simulink model "ros_image_filters_0619"  (R2017a)
settings: Solver=FixedStepDiscrete  StartTime=0.0  StopTime=inf  FixedStep=0.01  RelTol=1e-3  EnableMultiTasking=on
model workspace (MAT data in the model file):
  SL_ROS_VariableLengthArrays_MaxSizes.CommonInfo.ArrayTruncateAction = 'EmitWarning'
  SL_ROS_VariableLengthArrays_MaxSizes.MsgTypeMap = containers.Map
  SL_ROS_VariableLengthArrays_MaxSizes.MsgTypeMap.serialization.keys = {'sensor_msgs/Image'}
  SL_ROS_VariableLengthArrays_MaxSizes.MsgTypeMap.serialization.values{1}(1).PropertyName = 'Data'
  SL_ROS_VariableLengthArrays_MaxSizes.MsgTypeMap.serialization.values{1}(1).DataType = 'uint8'
  SL_ROS_VariableLengthArrays_MaxSizes.MsgTypeMap.serialization.values{1}(1).MaxLength = 1555200
  SL_ROS_VariableLengthArrays_MaxSizes.MsgTypeMap.serialization.values{1}(2).PropertyName = 'Encoding'
  SL_ROS_VariableLengthArrays_MaxSizes.MsgTypeMap.serialization.values{1}(2).DataType = 'uint8'
  SL_ROS_VariableLengthArrays_MaxSizes.MsgTypeMap.serialization.values{1}(2).MaxLength = 5
  SL_ROS_VariableLengthArrays_MaxSizes.MsgTypeMap.serialization.uniformity = 0
  SL_ROS_VariableLengthArrays_MaxSizes.MsgTypeMap.serialization.keyType = 'char'
  SL_ROS_VariableLengthArrays_MaxSizes.MsgTypeMap.serialization.valueType = 'any'
  blockSize = [270 480]
undefined symbols (not defined in the file): gray, M, N, Rec, SDTV, strel, sz
libraries: vipmisc x9, visionsinks x6, robotlib x5, visionconversions x4, simulink x3, visionanalysis x2, visionfilter x1, visionmorphops x1
settings Model: Creator=qifan  LastModifiedBy=qifan
settings SolverCC: AutoInsertRateTranBlk=on
settings DataIOCC: SaveOutput=off  SaveTime=off
settings OptimizationCC: PassReuseOutputArgsAs=Individual arguments  StateBitsets=on  DataBitsets=on  ZeroExternalMemoryAtStartup=off  ZeroInternalMemoryAtStartup=off  NoFixptDivByZeroProtection=on  LifeSpan=1  MaxStackSize=64
settings DebuggingCC: ParameterTunabilityLossMsg=error
settings HardwareCC: ProdBitPerPointer=32  ProdBitPerSizeT=32  ProdBitPerPtrDiffT=32  ProdLargestAtomicFloat=None  ProdIntDivRoundTo=Undefined  ProdEndianess=Unspecified  ProdWordSize=32  ProdHWDeviceType=Generic->Unspecified (assume 32-bit Generic)
settings SFSimCC: MATLABDynamicMemAlloc=off
settings RTWCC: SystemTargetFile=ert.tlc  HardwareBoard=Robot Operating System (ROS)  TLCOptions="-p0 -aInlineSetEventsForThisBaseRateFcn=TLC_FALSE -aSuppressMultiTaskScheduler=TLC_FALSE  -aRateBasedStepFcn=0"  GenCodeOnly=on  TemplateMakefile=ert_default_tmf  Description=Embedded Coder  GenerateReport=on  RTWVerbose=off  Toolchain=Catkin  IncludeHyperlinkInReport=on  LaunchReport=on  TargetLang=C++  GenerateTraceInfo=on  GenerateTraceReport=on  GenerateTraceReportSl=on  GenerateTraceReportSf=on  GenerateTraceReportEml=on
settings CodeAppCC: ForceParamTrailComments=on  IgnoreCustomStorageClasses=off  OperatorAnnotations=on  SimulinkDataObjDesc=on  SFDataObjDesc=on  MATLABFcnDesc=on  CustomSymbolStrGlobalVar=rt$N$M  CustomSymbolStrType=$N$M  CustomSymbolStrFcn=$N$M$F  CustomSymbolStrMacro=$N$M  InsertBlockDesc=on  MATLABSourceComments=on
settings ERTTargetCC: CodeReplacementLibrary=ISO_C  SuppressErrorStatus=on  SupportAbsoluteTime=off  SupportNonFinite=off  SupportComplex=off  RootIOFormat=Structure reference

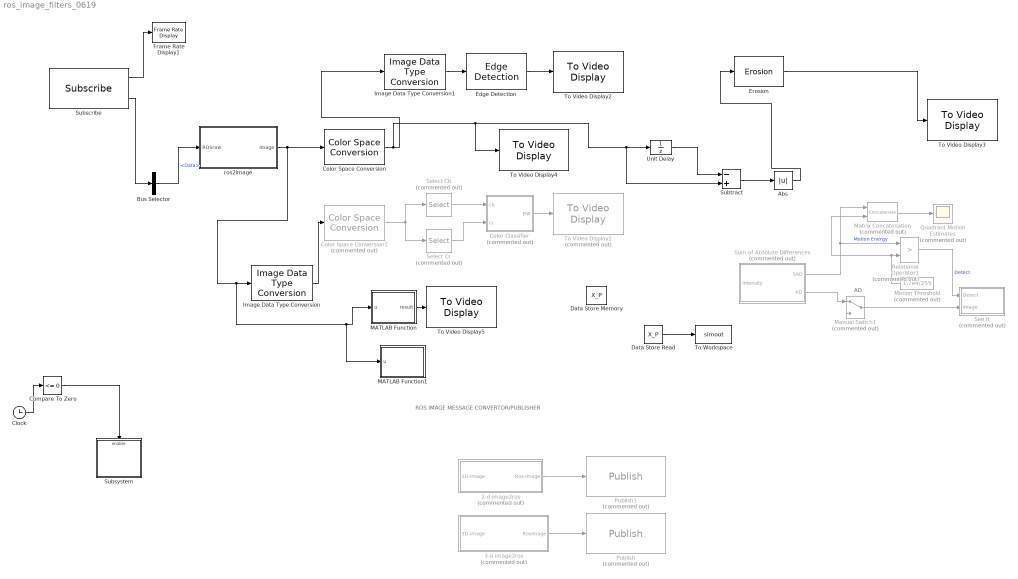
== system ros_image_filters_0619 ==
  note: ROS IMAGE MESSAGE CONVERTOR/PUBLISHER
  note: AD
  2-d-image2ros : Subsystem  Commented=on
  3-d-image2ros : Subsystem  Commented=on
  Abs : Abs
  Bus Selector : BusSelector  OutputSignals=Data
  Clock : Clock
  Color Classifier : Subsystem  Commented=on
  Color Space Conversion : visionconversions/Color Space  Conversion  conversion=Obsolete  conversionActive=R'G'B' to intensity  wp_str=D65  rec=Rec. 601 (SDTV)  sys=1125/60/2:1  imagePorts=One multidimensional signal
      settings: SourceProductName=Computer Vision System Toolbox
  Color Space Conversion1 : visionconversions/Color Space  Conversion  Commented=on  conversion=Obsolete  conversionActive=R'G'B' to Y'CbCr  wp_str=D65  rec=Rec. 601 (SDTV)  sys=1125/60/2:1  imagePorts=One multidimensional signal
      settings: SourceProductName=Computer Vision System Toolbox
  Compare To Zero : simulink/Logic and Bit Operations/Compare To Zero  relop=<=  OutDataTypeStr=boolean
  Data Store Memory : DataStoreMemory  DataStoreName=X_P  ReadBeforeWriteMsg=warning  WriteAfterWriteMsg=warning  WriteAfterReadMsg=warning  InitialValue=zeros(200,3,2)  ShowAdditionalParam=off  OutDataTypeStr=double
  Data Store Read : DataStoreRead  DataStoreName=X_P
  Edge Detection : visionanalysis/Edge Detection  method=Sobel  outputType=Binary image  userDefinedThreshold=off  thresholdSource=Input port  threshold=20  thresholdTuning=4  edgeThinning=off  threshold_canny=[0.25 0.60]  autoPercent=70  sigma=1  prodOutputMode=Binary point scaling  prodOutputWordLength=32  prodOutputFracLength=8  roundingMode=Floor  overflowMode=off
      settings: SourceProductName=Computer Vision System Toolbox  SourceProductBaseCode=VP
  Erosion : visionmorphops/Erosion  nhoodsrc=Specify via dialog  strel=strel('square',7)
      settings: SourceProductName=Computer Vision System Toolbox  SourceProductBaseCode=VP
  Frame Rate Display1 : visionsinks/Frame Rate Display  UpdateRate=10
      settings: SourceProductName=Computer Vision System Toolbox  SourceProductBaseCode=VP
  Image Data Type Conversion : visionconversions/Image Data Type Conversion  outDT=single  isSigned=on  wordLen=16  numFracBits=0
      settings: SourceProductName=Computer Vision System Toolbox  SourceProductBaseCode=VP
  Image Data Type Conversion1 : visionconversions/Image Data Type Conversion  outDT=single  isSigned=on  wordLen=16  numFracBits=0
      settings: SourceProductName=Computer Vision System Toolbox  SourceProductBaseCode=VP
  MATLAB Function : MATLAB Function  TreatAsAtomicUnit=on
  MATLAB Function1 : MATLAB Function  TreatAsAtomicUnit=on
  Manual Switch1 : ManualSwitch  Commented=on
  Matrix Concatenation : Concatenate  Commented=on  Mode=Multidimensional array
  Motion Threshold : Constant  Commented=on  Value=1.7e4/255  VectorParams1D=off  OutDataTypeStr=Inherit: Inherit via back propagation
  Publish : robotlib/Publish  Commented=on  SourceLibraryInfo=This block requires Robotics System Toolbox  topicSource=Specify your own  topic=/image_color  messageType=sensor_msgs/Image  messageQueueLength=1
      settings: SourceProductBaseCode=RO
  Publish1 : robotlib/Publish  Commented=on  SourceLibraryInfo=This block requires Robotics System Toolbox  topicSource=Specify your own  topic=/image_erode  messageType=sensor_msgs/Image  messageQueueLength=1
      settings: SourceProductBaseCode=RO
  Quadrant Motion Estimates : Scope  Commented=on
  Relational Operator1 : RelationalOperator  Commented=on  Operator=>  OutDataTypeStr=boolean  RndMeth=Nearest  InputSameDT=on
  See It : Subsystem  Commented=on
  Select Cb : Selector  Commented=on  NumberOfDimensions=3  InputPortWidth=3  IndexOptions=Select all,Select all,Index vector (dialog)  Indices=[1 3],1,2  OutputSizes=1,1,1
  Select Cr : Selector  Commented=on  NumberOfDimensions=3  InputPortWidth=3  IndexOptions=Select all,Select all,Index vector (dialog)  Indices=[1 3],1,3  OutputSizes=1,1,1
  Subscribe : robotlib/Subscribe  SourceLibraryInfo=This block requires Robotics System Toolbox  topicSource=Specify your own  topic=/image_bridge  messageType=sensor_msgs/Image  sampleTime=-1  messageQueueLength=1
      settings: SourceProductBaseCode=RO
  Subsystem : Subsystem
  Subtract : Sum  Inputs=-+
  Sum of Absolute Differences : Subsystem  Commented=on
  To Video Display1 : visionsinks/To Video Display  Commented=on  windowSizeMode=Normal  openAtMdlStart=on  fullScreen=off  videoWindowX=260  videoWindowY=97  saveWindowSize=off  videoWindowWidth=962  videoWindowHeight=542  inputColorFormat=RGB  inputType=Obsolete  imagePorts=One multidimensional signal  OutputDevice=On-screen video monitor  dataOrg=Column-major  isWindowOpen=off
      settings: SourceProductName=Computer Vision System Toolbox
  To Video Display2 : visionsinks/To Video Display  windowSizeMode=Normal  openAtMdlStart=on  fullScreen=off  videoWindowX=184  videoWindowY=153  saveWindowSize=off  videoWindowWidth=960  videoWindowHeight=540  inputColorFormat=RGB  inputType=Obsolete  imagePorts=One multidimensional signal  OutputDevice=On-screen video monitor  dataOrg=Column-major  isWindowOpen=off
      settings: SourceProductName=Computer Vision System Toolbox
  To Video Display3 : visionsinks/To Video Display  windowSizeMode=Normal  openAtMdlStart=on  fullScreen=off  videoWindowX=57  videoWindowY=109  saveWindowSize=off  videoWindowWidth=960  videoWindowHeight=540  inputColorFormat=RGB  inputType=Obsolete  imagePorts=One multidimensional signal  OutputDevice=On-screen video monitor  dataOrg=Column-major  isWindowOpen=off
      settings: SourceProductName=Computer Vision System Toolbox
  To Video Display4 : visionsinks/To Video Display  windowSizeMode=Normal  openAtMdlStart=on  fullScreen=off  videoWindowX=148  videoWindowY=171  saveWindowSize=off  videoWindowWidth=960  videoWindowHeight=540  inputColorFormat=RGB  inputType=Obsolete  imagePorts=One multidimensional signal  OutputDevice=On-screen video monitor  dataOrg=Column-major  isWindowOpen=off
      settings: SourceProductName=Computer Vision System Toolbox
  To Video Display5 : visionsinks/To Video Display  windowSizeMode=Normal  openAtMdlStart=on  fullScreen=off  videoWindowX=260  videoWindowY=97  saveWindowSize=off  videoWindowWidth=962  videoWindowHeight=542  inputColorFormat=RGB  inputType=Obsolete  imagePorts=One multidimensional signal  OutputDevice=On-screen video monitor  dataOrg=Column-major  isWindowOpen=off
      settings: SourceProductName=Computer Vision System Toolbox
  To Workspace : ToWorkspace  VariableName=simout  SaveFormat=Timeseries  SampleTime=-1
  Unit Delay : UnitDelay  SampleTime=-1
  ros2image : Subsystem
  wires:
  Subscribe/1 -> Frame Rate Display1/1
  Bus Selector/1 -> ros2image/1(ROSraw)  "<Data>"
  ros2image/1(Image) -> MATLAB Function1/1(u), MATLAB Function/1(u), Image Data Type Conversion/1, Color Space Conversion/1
  Subscribe/2 -> Bus Selector/1
  Color Space Conversion/1 -> To Video Display4/1, Subtract/2, Unit Delay/1, Image Data Type Conversion1/1
  3-d-image2ros/1(RosImage) -> Publish/1
  2-d-image2ros/1(Ros-image) -> Publish1/1
  Color Space Conversion1/1 -> Select Cr/1, Select Cb/1
  Select Cb/1 -> Color Classifier/1(cb)
  Select Cr/1 -> Color Classifier/2(cr)
  Color Classifier/1(BW) -> To Video Display1/1
  Image Data Type Conversion/1 -> Color Space Conversion1/1
  Edge Detection/1 -> To Video Display2/1
  Image Data Type Conversion1/1 -> Edge Detection/1
  Sum of Absolute Differences/1(SAD) -> Relational Operator1/1, Matrix Concatenation/1  "Motion Energy"
  Relational Operator1/1 -> See It/1(Detect)  "Detect"
  Motion Threshold/1 -> Relational Operator1/2, Matrix Concatenation/2
  Matrix Concatenation/1 -> Quadrant Motion Estimates/1
  Sum of Absolute Differences/2(AD) -> Manual Switch1/1
  Manual Switch1/1 -> See It/2(Image)
  Unit Delay/1 -> Subtract/1
  Subtract/1 -> Abs/1
  Abs/1 -> Erosion/1
  Erosion/1 -> To Video Display3/1
  MATLAB Function/1(result) -> To Video Display5/1
  Data Store Read/1 -> To Workspace/1
  Clock/1 -> Compare To Zero/1
  Compare To Zero/1 -> Subsystem/Enable

== system ros_image_filters_0619/2-d-image2ros ==
  2D-image : Inport
  2D_img_to_1D_img1 : MATLAB Function  TreatAsAtomicUnit=on
  Blank Message : robotlib/Blank Message  SourceLibraryInfo=This block requires Robotics System Toolbox  messageType=sensor_msgs/Image  SampleTime=inf
      settings: SourceProductBaseCode=RO
  ROS_Img_Data_to_ROS_Img1 : MATLAB Function  TreatAsAtomicUnit=on
  Ros-image : Outport
  wires:
  2D-image/1 -> 2D_img_to_1D_img1/1(data)
  ROS_Img_Data_to_ROS_Img1/1(y) -> Ros-image/1
  Blank Message/1 -> ROS_Img_Data_to_ROS_Img1/1(msg)
  2D_img_to_1D_img1/1(img) -> ROS_Img_Data_to_ROS_Img1/2(data)

== system ros_image_filters_0619/3-d-image2ros ==
  3D-image : Inport
  3D_img_to_1D_img : MATLAB Function  TreatAsAtomicUnit=on
  Blank Message : robotlib/Blank Message  SourceLibraryInfo=This block requires Robotics System Toolbox  messageType=sensor_msgs/Image  SampleTime=inf
      settings: SourceProductBaseCode=RO
  ROS_Img_Data_to_ROS_Img1 : MATLAB Function  TreatAsAtomicUnit=on
  RosImage : Outport
  wires:
  3D-image/1 -> 3D_img_to_1D_img/1(data)
  ROS_Img_Data_to_ROS_Img1/1(y) -> RosImage/1
  Blank Message/1 -> ROS_Img_Data_to_ROS_Img1/1(msg)
  3D_img_to_1D_img/1(img) -> ROS_Img_Data_to_ROS_Img1/2(data)

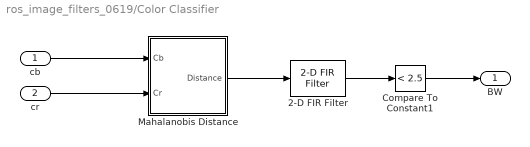
== system ros_image_filters_0619/Color Classifier ==
  cb : Inport
  cr : Inport  Port=2
  2-D FIR Filter : visionfilter/2-D FIR Filter  separable=off  filtSrc=Specify via dialog  filterMtrx=single(1/9*ones(3))  verticalFilter=[4 0]  horizontalFilter=[4 0]  outSize=Full  padType=Constant  padSrc=Specify via dialog  padVal=0  method=Convolution  firstCoeffSignedness=Signed  firstCoeffDataTypeStr=Inherit: Same word length as input  firstCoeffLastDataTypeStr=Inherit: Same word length as input  firstCoeffMin=[]  firstCoeffMax=[]  outputMode=Binary point scaling  outputWordLength=32  outputFracLength=12  outputSignedness=Auto  outputDataTypeStr=fixdt([],32,12)  outputLastDataTypeStr=fixdt([],32,12)  outputMin=[]  outputMax=[]  accumDataTypeStr=Inherit: Same as product output  accumLastDataTypeStr=Inherit: Same as product output  prodOutputMode=Binary point scaling  prodOutputWordLength=32  prodOutputFracLength=10  prodOutputDataTypeStr=fixdt([],32,10)  prodOutputLastDataTypeStr=fixdt([],32,10)  roundingMode=Floor  overflowMode=off
      settings: SourceProductName=Computer Vision System Toolbox  SourceProductBaseCode=VP
  Compare To Constant1 : simulink/Logic and Bit Operations/Compare To Constant  relop=<  const=2.5  OutDataTypeStr=boolean  ZeroCross=off
  "Mahalanobis Distance " : Subsystem
  BW : Outport
  wires:
  "Mahalanobis Distance "/1(Distance) -> 2-D FIR Filter/1
  cb/1 -> "Mahalanobis Distance "/1(Cb)
  cr/1 -> "Mahalanobis Distance "/2(Cr)
  Compare To Constant1/1 -> BW/1
  2-D FIR Filter/1 -> Compare To Constant1/1

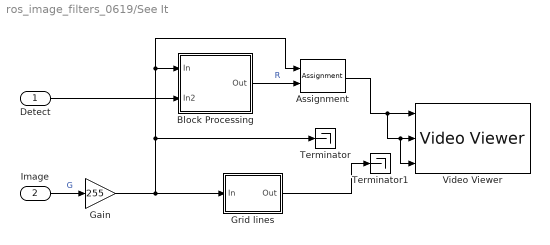
== system ros_image_filters_0619/See It ==
  Detect : Inport
  Image : Inport  Port=2
  Assignment : Assignment  NumberOfDimensions=2  IndexOptions=Starting index (dialog),Starting index (dialog)  Indices=1,1  OutputSizes=1,1
  Block Processing : Subsystem  DialogController=vipDDGCreate  TreatAsAtomicUnit=on  mask(Block Processing){NumI=2, ParamPort=off, NumO=1, Blocksize={blockSize, [1 1]}, Overlapsize={[0 0]}, Traverse=Row-wise}
      mask prompts: NumI "Number of inputs:"; ParamPort "Add port to supply subsystem parameters"; NumO "Number of outputs:"; Blocksize "Block size:"; Overlapsize "Overlap size:"; Traverse "Order of traversing:"
      mask help:
      | Repeats a user-specified operation on submatrices of the input matrix.
      |
      | This block extracts submatrices of a user-specified size from the input matrix. It sends each submatrix to a subsystem for processing, and then reassembles each subsystem output into the output matrix.
      |
      | Use the Block size and Overlap parameters to specify the size and overlap of each submatrix in cell array format.
      mask init:
      | errmsg = vipblkblockproc(gcbh, NumI, NumO, Blocksize, Overlapsize, Traverse, ParamPort);
      | error(errmsg);
      settings: CopyFcn=set_param(gcb,'LinkStatus','none');
      mask Help: eval('helpview(fullfile(docroot,''toolbox'',''vision'',''vision.map''),''vipblockprocessing'')');
      mask TypeOptions Traverse: Row-wise | Column-wise
      mask Display:
      | disp('Block\n Processing');
      | 
      | if ((NumI == 1) && ParamPort)
      |     port_label('input', 1, 'I');
      | end
      | 
      | if (NumI > 1)
      |     for (i = 1:NumI)
      |         port_label('input', i, ['I' int2str(i)]);
      |     end
      | end
      | 
      | if (ParamPort)
      |     port_label('input', NumI+1, 'P');
      | end
  Gain : Gain  Gain=255  OutDataTypeStr=uint(8)  ParamDataTypeStr=Inherit: Same as input
  Grid lines : Subsystem
  Terminator : Terminator
  Terminator1 : Terminator
  Video Viewer : VideoViewer  imagePorts=separate color signals  colormapValue=gray(256)  FigPos=[1 798 1223 678]
  wires:
  Image/1 -> Gain/1  "G"
  Detect/1 -> Block Processing/2(In2)
  Gain/1 -> Terminator/1, Assignment/1, Block Processing/1(In), Grid lines/1(In)
  Block Processing/1(Out) -> Assignment/2  "R"
  Assignment/1 -> Video Viewer/3, Video Viewer/2, Video Viewer/1
  Grid lines/1(Out) -> Terminator1/1

== system ros_image_filters_0619/Subsystem ==
  Enable : EnablePort
  MATLAB Function2 : MATLAB Function  TreatAsAtomicUnit=on

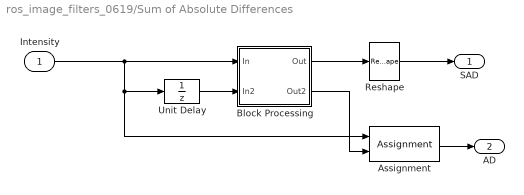
== system ros_image_filters_0619/Sum of Absolute Differences ==
  Intensity : Inport
  Assignment : Assignment  NumberOfDimensions=2  IndexOptions=Starting index (dialog),Starting index (dialog)  Indices=1,1  OutputSizes=1,1
  Block Processing : Subsystem  DialogController=vipDDGCreate  TreatAsAtomicUnit=on  mask(Block Processing){NumI=2, ParamPort=off, NumO=2, Blocksize={blockSize}, Overlapsize={[0 0]}, Traverse=Row-wise}
      mask prompts: NumI "Number of inputs:"; ParamPort "Add port to supply subsystem parameters"; NumO "Number of outputs:"; Blocksize "Block size:"; Overlapsize "Overlap size:"; Traverse "Order of traversing:"
      mask help:
      | Repeats a user-specified operation on submatrices of the input matrix.
      |
      | This block extracts submatrices of a user-specified size from the input matrix. It sends each submatrix to a subsystem for processing, and then reassembles each subsystem output into the output matrix.
      |
      | Use the Block size and Overlap parameters to specify the size and overlap of each submatrix in cell array format.
      mask init:
      | errmsg = vipblkblockproc(gcbh, NumI, NumO, Blocksize, Overlapsize, Traverse, ParamPort);
      | error(errmsg);
      settings: CopyFcn=set_param(gcb,'LinkStatus','none');
      mask Help: eval('helpview(fullfile(docroot,''toolbox'',''vision'',''vision.map''),''vipblockprocessing'')');
      mask TypeOptions Traverse: Row-wise | Column-wise
      mask Display:
      | disp('Block\n Processing');
      | 
      | if ((NumI == 1) && ParamPort)
      |     port_label('input', 1, 'I');
      | end
      | 
      | if (NumI > 1)
      |     for (i = 1:NumI)
      |         port_label('input', i, ['I' int2str(i)]);
      |     end
      | end
      | 
      | if (ParamPort)
      |     port_label('input', NumI+1, 'P');
      | end
  Reshape : Reshape  OutputDimensionality=Column vector (2-D)  OutputDimensions=[M,N]
  Unit Delay : UnitDelay  SampleTime=-1
  SAD : Outport
  AD : Outport  Port=2
  wires:
  Unit Delay/1 -> Block Processing/2(In2)
  Block Processing/1(Out) -> Reshape/1
  Reshape/1 -> SAD/1
  Intensity/1 -> Assignment/1, Unit Delay/1, Block Processing/1(In)
  Block Processing/2(Out2) -> Assignment/2
  Assignment/1 -> AD/1

== system ros_image_filters_0619/ros2image ==
  ROSraw : Inport  PortDimensions=1555200
  ROSraw2RGB : MATLAB Function  TreatAsAtomicUnit=on
  Reshape : Reshape  OutputDimensionality=Customize  OutputDimensions=[540,960,3]
  Vector Concatenate : Concatenate  NumInputs=3  Mode=Multidimensional array  ConcatenateDimension=2
  Image : Outport
  wires:
  ROSraw2RGB/3(B) -> Vector Concatenate/3
  ROSraw2RGB/1(R) -> Vector Concatenate/1
  Reshape/1 -> Image/1
  ROSraw/1 -> ROSraw2RGB/1(u)
  ROSraw2RGB/2(G) -> Vector Concatenate/2
  Vector Concatenate/1 -> Reshape/1

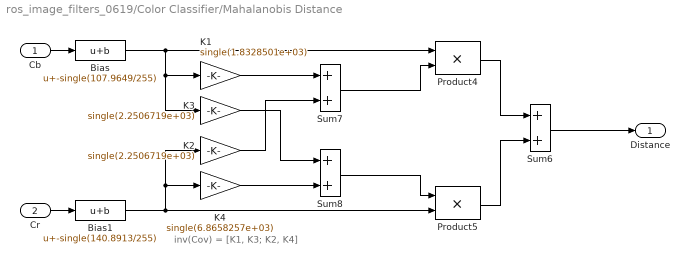
== system ros_image_filters_0619/Color Classifier/Mahalanobis Distance  ==
  note: inv(Cov) = [K1, K3; K2, K4]
  Cb : Inport
  Cr : Inport  Port=2
  Bias : Bias  Bias=-single(107.9649/255)
  Bias1 : Bias  Bias=-single(140.8913/255)
  K1 : Gain  Gain=single(1.8328501e+03)  SaturateOnIntegerOverflow=on  OutDataTypeStr=Inherit: Same as input  ParamDataTypeStr=Inherit: Same as input
  K2 : Gain  Gain=single(2.2506719e+03)  SaturateOnIntegerOverflow=on  OutDataTypeStr=Inherit: Same as input  ParamDataTypeStr=Inherit: Same as input
  K3 : Gain  Gain=single(2.2506719e+03)  SaturateOnIntegerOverflow=on  OutDataTypeStr=Inherit: Same as input  ParamDataTypeStr=Inherit: Same as input
  K4 : Gain  Gain=single(6.8658257e+03)  SaturateOnIntegerOverflow=on  OutDataTypeStr=Inherit: Same as input  ParamDataTypeStr=Inherit: Same as input
  Product4 : Product  SaturateOnIntegerOverflow=on  InputSameDT=on  OutDataTypeStr=Inherit: Same as first input
  Product5 : Product  SaturateOnIntegerOverflow=on  InputSameDT=on  OutDataTypeStr=Inherit: Same as first input
  Sum6 : Sum  SaturateOnIntegerOverflow=on  InputSameDT=on  OutDataTypeStr=Inherit: Same as first input
  Sum7 : Sum  SaturateOnIntegerOverflow=on  InputSameDT=on  OutDataTypeStr=Inherit: Same as first input
  Sum8 : Sum  SaturateOnIntegerOverflow=on  InputSameDT=on  OutDataTypeStr=Inherit: Same as first input
  Distance : Outport
  wires:
  Cb/1 -> Bias/1
  Cr/1 -> Bias1/1
  K4/1 -> Sum8/2
  Product4/1 -> Sum6/1
  Product5/1 -> Sum6/2
  K1/1 -> Sum7/1
  K2/1 -> Sum7/2
  K3/1 -> Sum8/1
  Sum7/1 -> Product4/2
  Sum8/1 -> Product5/1
  Bias/1 -> Product4/1, K1/1, K3/1
  Bias1/1 -> Product5/2, K4/1, K2/1
  Sum6/1 -> Distance/1

== system ros_image_filters_0619/See It/Block Processing ==
  In : Inport
  In2 : Inport  Port=2
  Block iterator : Subsystem
      settings: CopyFcn=set_param(gcb,'ReferenceBlock','');
  Iteration count : vipmisc/Iteration count  NumI=NumI  blksize=Blocksize  ovlpsize=Overlapsize
      settings: SourceProductName=Computer Vision System Toolbox  SourceProductBaseCode=VP
  Out : Outport
  wires:
  Iteration count/1 -> Block iterator/1(iter)
  In/1 -> Iteration count/1, Block iterator/2(In1)
  Block iterator/1(Out) -> Out/1
  In2/1 -> Block iterator/3(In2), Iteration count/2

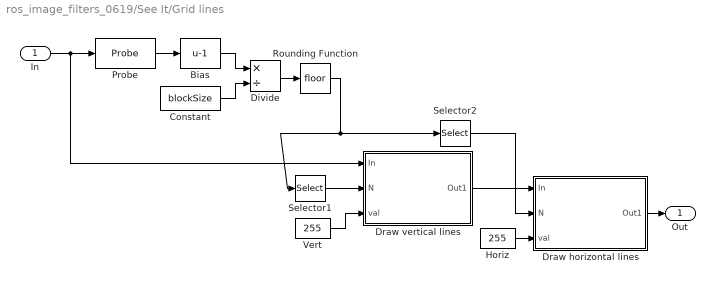
== system ros_image_filters_0619/See It/Grid lines ==
  In : Inport
  Bias : Bias  Bias=-1
  Constant : Constant  Value=blockSize
  Divide : Product  Inputs=*/
  Draw horizontal lines : Subsystem  TreatAsAtomicUnit=on
  Draw vertical lines : Subsystem  TreatAsAtomicUnit=on
  Horiz : Constant  Value=255  VectorParams1D=off  OutDataTypeStr=Inherit: Inherit via back propagation
  Probe : Probe  ProbeWidth=off  ProbeSampleTime=off  ProbeComplexSignal=off  ProbeSignalDimensions=on
  Rounding Function : Rounding
  Selector1 : Selector  InputPortWidth=2  IndexOptions=Index vector (dialog)  Indices=2  OutputSizes=1
  Selector2 : Selector  InputPortWidth=2  IndexOptions=Index vector (dialog)  Indices=1  OutputSizes=1
  Vert : Constant  Value=255  VectorParams1D=off  OutDataTypeStr=Inherit: Inherit via back propagation
  Out : Outport
  wires:
  In/1 -> Probe/1, Draw vertical lines/1(In)
  Probe/1 -> Bias/1
  Bias/1 -> Divide/1
  Constant/1 -> Divide/2
  Divide/1 -> Rounding Function/1
  Selector1/1 -> Draw vertical lines/2(N)
  Rounding Function/1 -> Selector1/1, Selector2/1
  Vert/1 -> Draw vertical lines/3(val)
  Draw vertical lines/1(Out1) -> Draw horizontal lines/1(In)
  Selector2/1 -> Draw horizontal lines/2(N)
  Horiz/1 -> Draw horizontal lines/3(val)
  Draw horizontal lines/1(Out1) -> Out/1

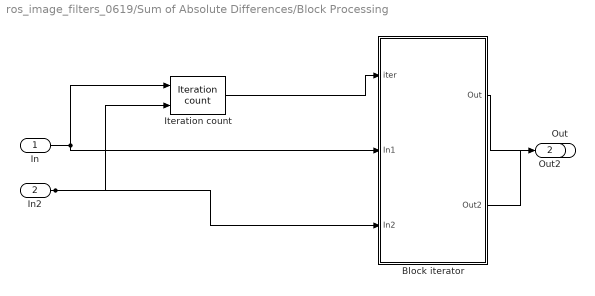
== system ros_image_filters_0619/Sum of Absolute Differences/Block Processing ==
  In : Inport
  In2 : Inport  Port=2
  Block iterator : Subsystem
      settings: CopyFcn=set_param(gcb,'ReferenceBlock','');
  Iteration count : vipmisc/Iteration count  NumI=NumI  blksize=Blocksize  ovlpsize=Overlapsize
      settings: SourceProductName=Computer Vision System Toolbox  SourceProductBaseCode=VP
  Out : Outport
  Out2 : Outport  Port=2
  wires:
  Iteration count/1 -> Block iterator/1(iter)
  In/1 -> Iteration count/1, Block iterator/2(In1)
  Block iterator/1(Out) -> Out/1
  In2/1 -> Block iterator/3(In2), Iteration count/2
  Block iterator/2(Out2) -> Out2/1

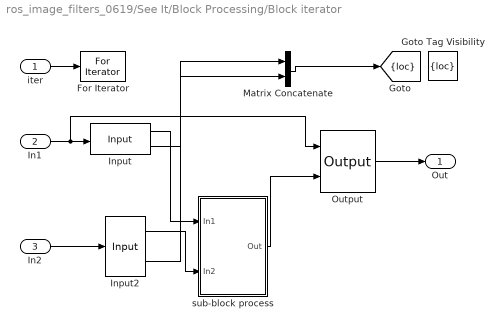
== system ros_image_filters_0619/See It/Block Processing/Block iterator ==
  iter : Inport
  In1 : Inport  Port=2
  In2 : Inport  Port=3
  For Iterator : ForIterator  IterationSource=external  IterationLimit=(sz(1)/M)*(sz(2)/N)  ShowIterationPort=off  IndexMode=Zero-based  IterationVariableDataType=double
  Goto Tag Visibility : GotoTagVisibility  GotoTag=loc
  Input : vipmisc/Input  Blocksize=Blocksize{1}  Overlapsize=Overlapsize{1}  tverse=Row-wise
      settings: SourceProductName=Computer Vision System Toolbox  SourceProductBaseCode=VP
  Input2 : vipmisc/Input  Blocksize=Blocksize{2}  Overlapsize=Overlapsize{1}  tverse=Row-wise
      settings: SourceProductName=Computer Vision System Toolbox  SourceProductBaseCode=VP
  Matrix Concatenate : Concatenate  Mode=Multidimensional array  ConcatenateDimension=2
  Output : vipmisc/Output  Blocksize=Blocksize{1}  Overlapsize=Overlapsize{1}  tverse=Row-wise
      settings: SourceProductName=Computer Vision System Toolbox  SourceProductBaseCode=VP
  sub-block process : Subsystem
  Out : Outport
  tag scope: loc=scoped
  wires:
  Matrix Concatenate/1 -> [loc]
  Input/2 -> Matrix Concatenate/1
  Input/1 -> sub-block process/1(In1)
  iter/1 -> For Iterator/1
  In1/1 -> Input/1, Output/1
  Output/1 -> Out/1
  sub-block process/1(Out) -> Output/2
  Input2/2 -> Matrix Concatenate/2
  In2/1 -> Input2/1
  Input2/1 -> sub-block process/2(In2)

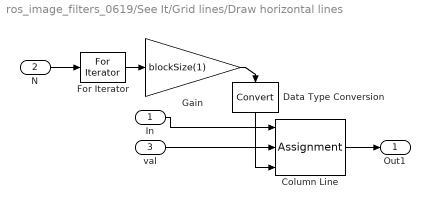
== system ros_image_filters_0619/See It/Grid lines/Draw horizontal lines ==
  In : Inport
  N : Inport  Port=2
  val : Inport  Port=3
  Column Line : Assignment  NumberOfDimensions=2  IndexOptions=Index vector (port),Assign all  Indices=60,-1  OutputSizes=1,1
  Data Type Conversion : DataTypeConversion
  For Iterator : ForIterator  IterationSource=external
  Gain : Gain  Gain=blockSize(1)
  Out1 : Outport
  wires:
  Data Type Conversion/1 -> Column Line/3
  Gain/1 -> Data Type Conversion/1
  val/1 -> Column Line/2
  In/1 -> Column Line/1
  Column Line/1 -> Out1/1
  For Iterator/1 -> Gain/1
  N/1 -> For Iterator/1

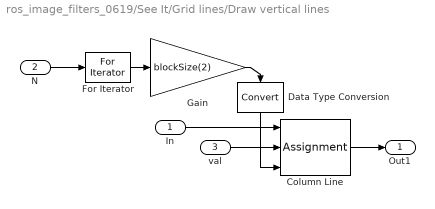
== system ros_image_filters_0619/See It/Grid lines/Draw vertical lines ==
  In : Inport
  N : Inport  Port=2
  val : Inport  Port=3
  Column Line : Assignment  NumberOfDimensions=2  IndexOptions=Assign all,Index vector (port)  Indices=60,-1  OutputSizes=1,1
  Data Type Conversion : DataTypeConversion
  For Iterator : ForIterator  IterationSource=external
  Gain : Gain  Gain=blockSize(2)
  Out1 : Outport
  wires:
  N/1 -> For Iterator/1
  For Iterator/1 -> Gain/1
  Column Line/1 -> Out1/1
  In/1 -> Column Line/1
  val/1 -> Column Line/2
  Gain/1 -> Data Type Conversion/1
  Data Type Conversion/1 -> Column Line/3

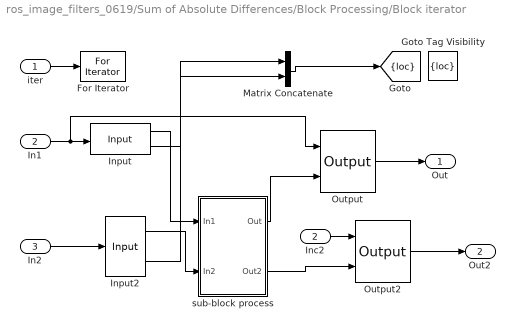
== system ros_image_filters_0619/Sum of Absolute Differences/Block Processing/Block iterator ==
  iter : Inport
  In1 : Inport  Port=2
  In2 : Inport  Port=3
  For Iterator : ForIterator  IterationSource=external  IterationLimit=(sz(1)/M)*(sz(2)/N)  ShowIterationPort=off  IndexMode=Zero-based  IterationVariableDataType=double
  Goto Tag Visibility : GotoTagVisibility  GotoTag=loc
  Inc2 : InportShadow  Port=2
  Input : vipmisc/Input  Blocksize=Blocksize{1}  Overlapsize=Overlapsize{1}  tverse=Row-wise
      settings: SourceProductName=Computer Vision System Toolbox  SourceProductBaseCode=VP
  Input2 : vipmisc/Input  Blocksize=Blocksize{1}  Overlapsize=Overlapsize{1}  tverse=Row-wise
      settings: SourceProductName=Computer Vision System Toolbox  SourceProductBaseCode=VP
  Matrix Concatenate : Concatenate  Mode=Multidimensional array  ConcatenateDimension=2
  Output : vipmisc/Output  Blocksize=Blocksize{1}  Overlapsize=Overlapsize{1}  tverse=Row-wise
      settings: SourceProductName=Computer Vision System Toolbox  SourceProductBaseCode=VP
  Output2 : vipmisc/Output  Blocksize=Blocksize{1}  Overlapsize=Overlapsize{1}  tverse=Row-wise
      settings: SourceProductName=Computer Vision System Toolbox  SourceProductBaseCode=VP
  sub-block process : Subsystem
  Out : Outport
  Out2 : Outport  Port=2
  tag scope: loc=scoped
  wires:
  Matrix Concatenate/1 -> [loc]
  Input/2 -> Matrix Concatenate/1
  Input/1 -> sub-block process/1(In1)
  iter/1 -> For Iterator/1
  In1/1 -> Input/1, Output/1
  Output/1 -> Out/1
  sub-block process/1(Out) -> Output/2
  Input2/2 -> Matrix Concatenate/2
  In2/1 -> Input2/1
  Input2/1 -> sub-block process/2(In2)
  Inc2/1 -> Output2/1
  Output2/1 -> Out2/1
  sub-block process/2(Out2) -> Output2/2

== system ros_image_filters_0619/See It/Block Processing/Block iterator/sub-block process ==
  note: To avoid unexpected behavior from the mask
      | callback function, do not rename input and output ports or
      | remove the From block.
  note: Place your block
      | processing system here.
  In1 : Inport
  In2 : Inport  Port=2
  Subsystem2 : Subsystem
  Terminator I : Terminator
  Out : Outport
  wires:
  [loc] -> Terminator I/1
  In2/1 -> Subsystem2/2(Sw)
  Subsystem2/1(Out) -> Out/1
  In1/1 -> Subsystem2/1(Quad)

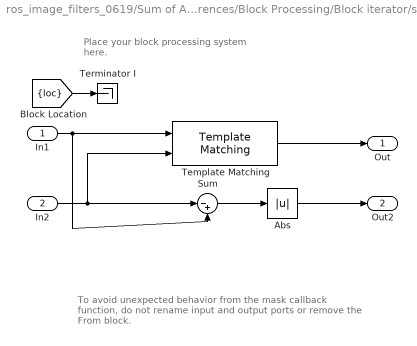
== system ros_image_filters_0619/Sum of Absolute Differences/Block Processing/Block iterator/sub-block process ==
  note: To avoid unexpected behavior from the mask
      | callback function, do not rename input and output ports or
      | remove the From block.
  note: Place your block
      | processing system here.
  In1 : Inport
  In2 : Inport  Port=2
  Abs : Abs  SaturateOnIntegerOverflow=on
  Sum : Sum  Inputs=|-+
  Template Matching : visionanalysis/Template Matching  metric=Sum of absolute differences  output=Metric matrix  method=Exhaustive  nMetric=off  nSize=3  roi=off  roiValid=off  accumMode=Binary point scaling  accumWordLength=32  accumFracLength=0  prodOutputMode=Binary point scaling  prodOutputWordLength=32  prodOutputFracLength=0  roundingMode=Floor  overflowMode=off
      settings: SourceProductName=Computer Vision System Toolbox  SourceProductBaseCode=VP
  Terminator I : Terminator
  Out : Outport
  Out2 : Outport  Port=2
  wires:
  [loc] -> Terminator I/1
  Template Matching/1 -> Out/1
  Abs/1 -> Out2/1
  Sum/1 -> Abs/1
  In2/1 -> Sum/1, Template Matching/2
  In1/1 -> Sum/2, Template Matching/1

== system ros_image_filters_0619/See It/Block Processing/Block iterator/sub-block process/Subsystem2 ==
  Quad : Inport
  Sw : Inport  Port=2
  Bitwise Logical Operator : simulink/Logic and Bit Operations/Bitwise Operator  logicop=XOR  UseBitMask=on  BitMask='FF'  BitMaskRealWorld=Stored Integer
  Switch : Switch  Criteria=u2 ~= 0  SaturateOnIntegerOverflow=on  InputSameDT=on
  Out : Outport
  wires:
  Quad/1 -> Switch/3, Bitwise Logical Operator/1
  Bitwise Logical Operator/1 -> Switch/1
  Sw/1 -> Switch/2
  Switch/1 -> Out/1

== matlab function ros_image_filters_0619/3-d-image2ros/ROS_Img_Data_to_ROS_Img1 ==
  data: msg input; y output Bus: SL_Bus_ros_image_filters_0619_sensor_msgs_Image; data input size=1555200
function y = rosImgData2rosImg(msg, data)
% assignString - Assign a string in a ROS message
%
% MSG = assignString(blankMsg) assigns a known string value to a 
%  string field in a ROS message, and outputs the updated ROS message.
%
%  blankMsg (input): A bus for a 'std_msgs/String' message. This is 
%      used to initialize the output. 
%  msg (output): A bus for a 'std_msgs/String' message, with the Data 
%      field set to a string.

%   Copyright 2015 The MathWorks, Inc.
%#codegen

% Note: The datatype of 'msg' has been explicitly set to the appropriate 
% Simulink bus type ("Bus: SL_Bus_robotROSMessageUsageExample_std_msgs_String"). 
%
% If the model name is changed, the datatype needs to be changed as well:
%   1) Click "Edit Data" in the Editor toolstrip to open "Ports and Data Manager"
%   2) Select "msg". From the "Type" dropdown, select "--- Refresh data types ---"
%   3) Set datatype to "Bus: SL_Bus_<modelname>_std_msgs_String"
    
stringToAssign = 'rgb8';
height = 540;
width = 960;

% msg (std_msgs/String) consists of
%           Data : array of type uint8
%   Data_SL_Info : struct with fields CurrentLength, ReceivedLength
msg.Encoding = uint8(stringToAssign)';
msg.Encoding_SL_Info.CurrentLength = uint32(length(stringToAssign));

msg.Data = uint8(data);
msg.Data_SL_Info.CurrentLength = uint32(length(data));

msg.Height = uint32(height);
msg.Width = uint32(width);
msg.Step = uint32(width * 3);

y = msg;

== matlab function ros_image_filters_0619/3-d-image2ros/3D_img_to_1D_img ==
  data: img output uint8; data input
function img = threeD_img_to_1D_img(data)
% assignString - Assign a string in a ROS message
%
% MSG = assignString(blankMsg) assigns a known string value to a 
%  string field in a ROS message, and outputs the updated ROS message.
%
%  blankMsg (input): A bus for a 'std_msgs/String' message. This is 
%      used to initialize the output. 
%  msg (output): A bus for a 'std_msgs/String' message, with the Data 
%      field set to a string.

%   Copyright 2015 The MathWorks, Inc.
%#codegen

% Note: The datatype of 'msg' has been explicitly set to the appropriate 
% Simulink bus type ("Bus: SL_Bus_robotROSMessageUsageExample_std_msgs_String"). 
%
% If the model name is changed, the datatype needs to be changed as well:
%   1) Click "Edit Data" in the Editor toolstrip to open "Ports and Data Manager"
%   2) Select "msg". From the "Type" dropdown, select "--- Refresh data types ---"
%   3) Set datatype to "Bus: SL_Bus_<modelname>_std_msgs_String"
    

% msg (std_msgs/String) consists of
%           Data : array of type uint8
%   Data_SL_Info : struct with fields CurrentLength, ReceivedLength
img = uint8(zeros(1, 1555200));
img(1:3:end) = data(:,:,1)';
img(2:3:end) = data(:,:,2)';
img(3:3:end) = data(:,:,3)';

== matlab function ros_image_filters_0619/MATLAB Function ==
  data: u input; result output
function result = fcn(u)

R = u(:, :, 1);
G = u(:, :, 2);
B = u(:, :, 3);


result = zeros(540, 960, 3);

result(:, :, 1) = R./(R + G + B);
result(:, :, 2) = G./(R + G + B);
result(:, :, 3) = B./(R + G + B);

%{
for i = 1:540
    for j = 1:960
        rgb = u(i, j, :);
        if rgb(1) > 95 && rgb(2) > 40 && rgb(3) > 20 && max(rgb) - min(rgb) > 15 ...
            && abs(rgb(1) - rgb(2)) > 15 && rgb(1) > rgb(2) && rgb(1) > rgb(3)
            result(i, j) = 255;
        end
    end
end
%}

== matlab function ros_image_filters_0619/2-d-image2ros/2D_img_to_1D_img1 ==
  data: img output uint8; data input
function img = twoD_img_to_1D_img(data)
% assignString - Assign a string in a ROS message
%
% MSG = assignString(blankMsg) assigns a known string value to a 
%  string field in a ROS message, and outputs the updated ROS message.
%
%  blankMsg (input): A bus for a 'std_msgs/String' message. This is 
%      used to initialize the output. 
%  msg (output): A bus for a 'std_msgs/String' message, with the Data 
%      field set to a string.

%   Copyright 2015 The MathWorks, Inc.
%#codegen

% Note: The datatype of 'msg' has been explicitly set to the appropriate 
% Simulink bus type ("Bus: SL_Bus_robotROSMessageUsageExample_std_msgs_String"). 
%
% If the model name is changed, the datatype needs to be changed as well:
%   1) Click "Edit Data" in the Editor toolstrip to open "Ports and Data Manager"
%   2) Select "msg". From the "Type" dropdown, select "--- Refresh data types ---"
%   3) Set datatype to "Bus: SL_Bus_<modelname>_std_msgs_String"
    

% msg (std_msgs/String) consists of
%           Data : array of type uint8
%   Data_SL_Info : struct with fields CurrentLength, ReceivedLength
img = uint8(zeros(1, 1555200));
img(1:3:end) = data';
img(2:3:end) = data';
img(3:3:end) = data';

== matlab function ros_image_filters_0619/2-d-image2ros/ROS_Img_Data_to_ROS_Img1 ==
  data: msg input; y output Bus: SL_Bus_ros_image_filters_0619_sensor_msgs_Image; data input size=1555200
function y = rosImgData2rosImg(msg, data)
% assignString - Assign a string in a ROS message
%
% MSG = assignString(blankMsg) assigns a known string value to a 
%  string field in a ROS message, and outputs the updated ROS message.
%
%  blankMsg (input): A bus for a 'std_msgs/String' message. This is 
%      used to initialize the output. 
%  msg (output): A bus for a 'std_msgs/String' message, with the Data 
%      field set to a string.

%   Copyright 2015 The MathWorks, Inc.
%#codegen

% Note: The datatype of 'msg' has been explicitly set to the appropriate 
% Simulink bus type ("Bus: SL_Bus_robotROSMessageUsageExample_std_msgs_String"). 
%
% If the model name is changed, the datatype needs to be changed as well:
%   1) Click "Edit Data" in the Editor toolstrip to open "Ports and Data Manager"
%   2) Select "msg". From the "Type" dropdown, select "--- Refresh data types ---"
%   3) Set datatype to "Bus: SL_Bus_<modelname>_std_msgs_String"
    
stringToAssign = 'rgb8';
height = 540;
width = 960;

% msg (std_msgs/String) consists of
%           Data : array of type uint8
%   Data_SL_Info : struct with fields CurrentLength, ReceivedLength
msg.Encoding = uint8(stringToAssign)';
msg.Encoding_SL_Info.CurrentLength = uint32(length(stringToAssign));

msg.Data = uint8(data);
msg.Data_SL_Info.CurrentLength = uint32(length(data));

msg.Height = uint32(height);
msg.Width = uint32(width);
msg.Step = uint32(width * 3);

y = msg;

== matlab function ros_image_filters_0619/ros2image/ROSraw2RGB ==
  data: u input; R output; G output; B output
function [R,G,B] = fcn(u)
%#codegen
Rs = u(1:3:end);
Gs = u(2:3:end);
Bs = u(3:3:end);
B = reshape(Rs,960,540)';
G = reshape(Gs,960,540)';
R = reshape(Bs,960,540)';

== matlab function ros_image_filters_0619/MATLAB Function1 ==
  data: u input; X_P data_store_memory
function fcn(u)

global X_P;

N = 200;
W = 50;
V = 0;

for i = 1:200
    X_P(i,:,:) = [8,8;8,8;8,8];
end

== matlab function ros_image_filters_0619/Subsystem/MATLAB Function2 ==
  data: X_P data_store_memory
function fcn

global X_P;

for i = 1:200
    X_P(i,2,:) = [0, 0];
    X_P(i,3,:) = [30, 30];
    x = rand * 960;
    y = rand * 540;
    X_P(i,1,:) = [x, y];
    
    
end
